simulink subsystem "Environment_Model"  (R2020b)
settings: Solver=VariableStepAuto  StartTime=0.0  StopTime=10.0  RelTol=1e-3
libraries: aerolibatmos2 x1, aerolibconvert2 x1
settings Model: Creator=Fatih  LastModifiedBy=Fatih

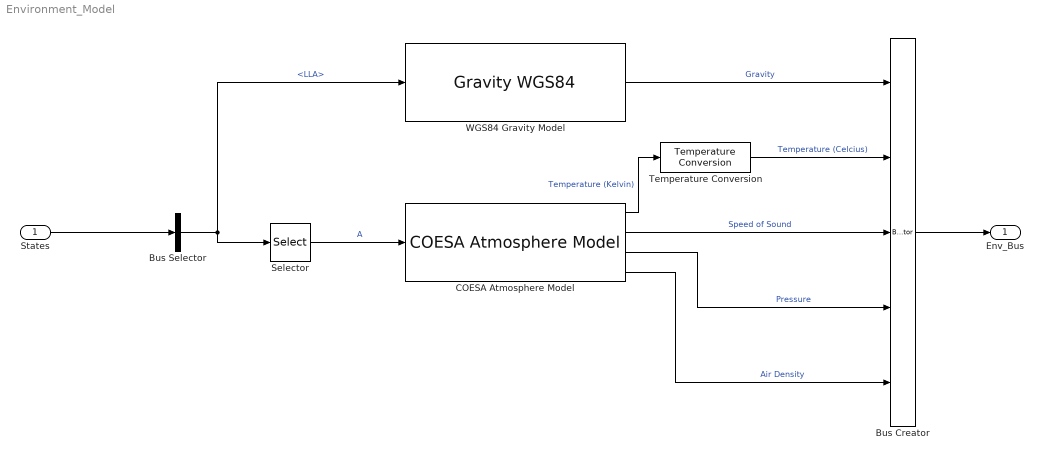
== system Environment_Model ==
  States : Inport
  Bus Creator : BusCreator  Inputs=5
  Bus Selector : BusSelector  OutputSignals=LLA
  COESA Atmosphere Model : aerolibatmos2/COESA Atmosphere Model  units=Metric (MKS)  spec=1976 COESA-extended U.S. Standard Atmosphere  model=Profile  profile_var=High temperature  profile_percent=1%  profile_alt=5 km (16404 ft)  envelope_var=High temperature  envelope_percent=1%  action=Warning
  Selector : Selector  InputPortWidth=3  IndexOptions=Index vector (dialog)  Indices=[3]  OutputSizes=1
  Temperature Conversion : aerolibconvert2/Temperature Conversion  IU=K  OU=C
      settings: SourceProductBaseCode=AE
  "WGS84 Gravity Model  " : GravityWGS84
  Env_Bus : Outport
  wires:
  "WGS84 Gravity Model  "/1 -> Bus Creator/1  "Gravity"
  COESA Atmosphere Model/1 -> Temperature Conversion/1  "Temperature (Kelvin)"
  COESA Atmosphere Model/2 -> Bus Creator/3  "Speed of Sound"
  COESA Atmosphere Model/3 -> Bus Creator/4  "Pressure"
  COESA Atmosphere Model/4 -> Bus Creator/5  "Air Density"
  Temperature Conversion/1 -> Bus Creator/2  "Temperature (Celcius)"
  Bus Creator/1 -> Env_Bus/1
  Selector/1 -> COESA Atmosphere Model/1  "A"
  States/1 -> Bus Selector/1
  Bus Selector/1 -> Selector/1, "WGS84 Gravity Model  "/1  "<LLA>"
